simulink model "simulink_elevation_model"  (R2021b)
settings: Solver=FixedStepAuto  StartTime=0.0  StopTime=6  RelTol=1e-3
values from neighbouring files (symbols this model uses):
  fric_gear_motor = 0.0226    [loading_project.m]
  fric_gear_turrent_gun = 100/(185)    (= 0.540540540541)    [loading_project.m]
  ts3 = 10^-3    (= 0.001)    [loading_project.m]
libraries: simulink x4, dspsrcs4 x1
(part 1 of 2)
settings Model: Creator=noait  LastModifiedBy=noait

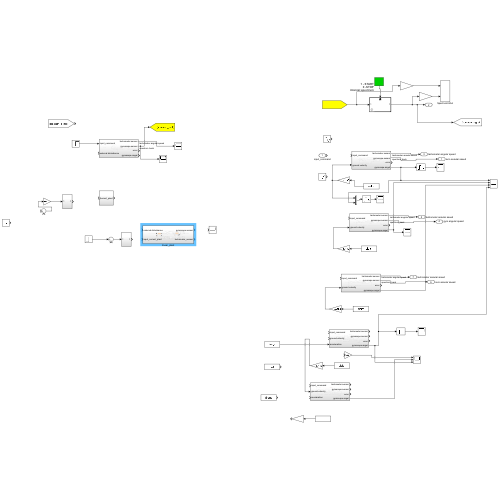
[thumbnail: Simulink's stored preview of the top-level diagram]
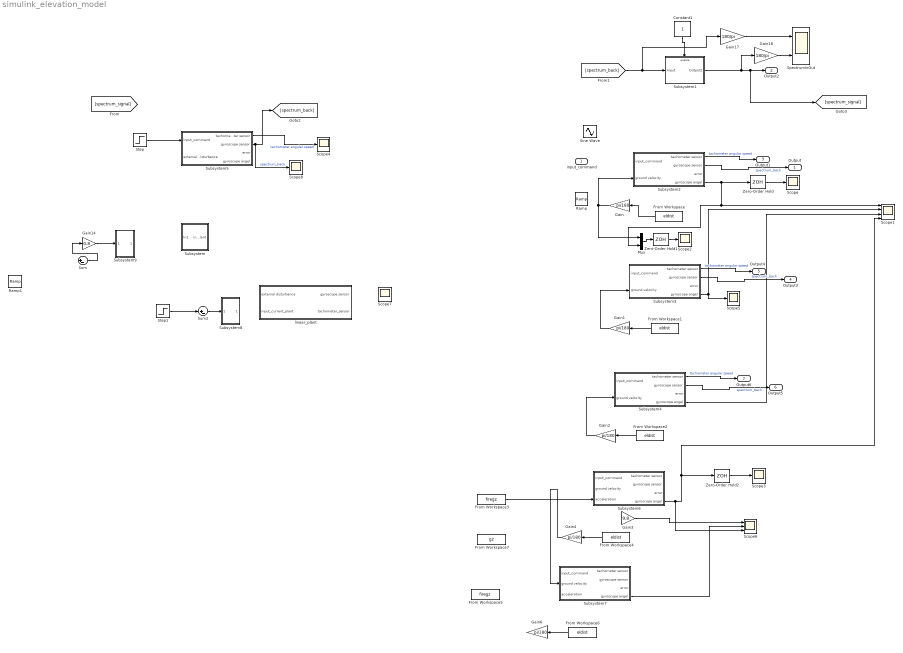
== system simulink_elevation_model ==
  input_command : Inport
  Constant1 : Constant  OutDataTypeStr=boolean
      settings: AttributesFormatString=1 - START\n0 -STOP\ninternal spectrum
      settings: OpenFcn=|
      | if get_param(gcbh,'value')-48 set_param(gcbh,'value','0','backgroundcolor','red');
      | else set_param(gcbh,'value','1','backgroundcolor','green');
      | end
  From Workspace{,1..2,4,6} (5 alike) : FromWorkspace  VariableName=eldist  SampleTime=-1  Interpolate=off  ZeroCross=off  OutputAfterFinalValue=Setting to zero
  From Workspace3 : FromWorkspace  VariableName=firegz  SampleTime=-1  OutputAfterFinalValue=Setting to zero
  From Workspace5 : FromWorkspace  VariableName=firegz  SampleTime=-1  OutputAfterFinalValue=Setting to zero
  From Workspace7 : FromWorkspace  VariableName=gz  SampleTime=ts3/3
  Gain{,1..2,4,6} (5 alike) : Gain  Gain=pi/180
  Gain14 : Gain  Gain=0.8
  Gain17 : Gain  Gain=180/pi
  Gain18 : Gain  Gain=180/pi
  Gain3 : Gain  Gain=9.8
  Mux : Mux  Inputs=2
  Ramp : simulink/Sources/Ramp  slope=1  start=0  InitialOutput=0
  Ramp1 : simulink/Sources/Ramp  slope=1  start=0  InitialOutput=0
  Scope{,2..5,7..8} (7 alike) : Scope
  Scope1 : Scope  NumInputPorts=4
  Scope6 : Scope  NumInputPorts=3
  Sine Wave : Sin  Amplitude=0.05  Frequency=2*pi  SampleTime=0
  SpectrumInOut : Scope  NumInputPorts=2
  Step : Step  After=0.05  SampleTime=0  VectorParams1D=off  ZeroCross=off
  Step1 : Step  SampleTime=0  ZeroCross=off
  Subsystem : Subsystem
  Subsystem1 : Subsystem  mask{GAIN=0.05%2*pi/180%0.5*pi/180, InitFreq=1, TargetTime=500, FreqAtTime=500}
      mask prompts: InitFreq "INITIAL FREQUENCY"; TargetTime "Target Time"; FreqAtTime "Frequency at Time"
  Subsystem2 : Subsystem
  Subsystem3 : Subsystem
  Subsystem4 : Subsystem
  Subsystem5 : Subsystem
  Subsystem6 : Subsystem
  Subsystem7 : Subsystem
  Subsystem8 : Subsystem
  Subsystem9 : Subsystem
  Sum : Sum  Inputs=|+-
  Sum2 : Sum  Inputs=|+-
  Zero-Order Hold : ZeroOrderHold  SampleTime=-1
  Zero-Order Hold1 : ZeroOrderHold  SampleTime=-1
  Zero-Order Hold2 : ZeroOrderHold  SampleTime=-1
  linear_plant : Subsystem  Description=elevation-plant
  Output : Outport  SignalName=gyro angular speed
  Output2 : Outport  Port=2
  Output1 : Outport  Port=3  SignalName=tachometer angular speed
  Output3 : Outport  Port=4  SignalName=gyro angular speed
  Output4 : Outport  Port=5  SignalName=tachometer angular speed
  Output5 : Outport  Port=6  SignalName=gyro angular speed
  Output6 : Outport  Port=7  SignalName=tachometer angular speed
  wires:
  Subsystem2/1(tachometer sensor) -> Output1/1  "tachometer angular speed"
  Gain18/1 -> SpectrumInOut/2
  Subsystem1/1(Output2) -> [spectrum_signal], Output2/1, Gain18/1
  Gain17/1 -> SpectrumInOut/1
  [spectrum_back] -> Gain17/1, Subsystem1/1(Input)
  Subsystem2/2(gyroscope sensor) -> Output/1  "spectrum_back"
  Constant1/1 -> Subsystem1/Enable
  Gain/1 -> Subsystem2/2(ground velocity), Mux/1
  Subsystem3/2(gyroscope sensor) -> Output3/1  "spectrum_back"
  From Workspace1/1 -> Gain1/1
  Gain1/1 -> Subsystem3/2(ground velocity)
  Subsystem3/1(tachometer sensor) -> Output4/1  "tachometer angular speed"
  Subsystem3/4(gyroscope angel) -> Scope5/1, Scope1/2
  Subsystem4/1(tachometer sensor) -> Output6/1  "tachometer angular speed"
  From Workspace2/1 -> Gain2/1
  Gain2/1 -> Subsystem4/2(ground velocity)
  Subsystem4/2(gyroscope sensor) -> Output5/1  "spectrum_back"
  Subsystem4/4(gyroscope angel) -> Scope1/3
  From Workspace/1 -> Gain/1
  Subsystem2/4(gyroscope angel) -> Zero-Order Hold/1, Mux/2, Scope1/1
  Zero-Order Hold/1 -> Scope/1
  Zero-Order Hold1/1 -> Scope2/1
  Mux/1 -> Zero-Order Hold1/1
  From Workspace4/1 -> Gain4/1
  Gain3/1 -> Scope6/1
  Subsystem7/4(gyroscope angel) -> Scope6/2
  From Workspace6/1 -> Gain6/1
  Sum/1 -> Gain14/1
  Gain14/1 -> Subsystem9/1(In1)
  Zero-Order Hold2/1 -> Scope3/1
  Subsystem6/4(gyroscope angel) -> Scope6/3, Zero-Order Hold2/1, Scope1/4
  Subsystem5/1(tachometer sensor) -> Scope4/1  "tachometer angular speed"
  Gain4/1 -> Subsystem7/2(ground velocity)
  From Workspace3/1 -> Subsystem6/3(acceleration)
  Sum2/1 -> Subsystem8/1(In1)
  Step1/1 -> Sum2/1
  Step/1 -> Subsystem5/1(input_command)
  Subsystem5/2(gyroscope sensor) -> Scope8/1, [spectrum_back]  "spectrum_back"

== system simulink_elevation_model/Subsystem ==
  In1 : Inport
  Gain : Gain  Gain=4.5
  Gain1 : Gain
  Gain2 : Gain  Gain=1.8*2*pi
  Integrator : Integrator
  Sum : Sum  Inputs=|++
  Transfer Fcn1 : TransferFcn  Numerator=[1 21 1.806*10^4]  Denominator=[1 25.035 2.102*10^4]
  Transfer Fcn10 : TransferFcn  Numerator=[1 59.495 9.908*10^4]  Denominator=[1 40 8.72*10^4]
  Transfer Fcn7 : TransferFcn  Denominator=[1/(2*pi*6.38)^2 0.55/355 1]
  Transfer Fcn8 : TransferFcn  Numerator=[1 2*0.08*2*35.6*pi (2*pi*35.6)^2]  Denominator=[1 2*0.94*2*35.6*pi (2*pi*35.6)^2]
  input_current_plant : Outport
  wires:
  In1/1 -> Transfer Fcn7/1
  Transfer Fcn8/1 -> Gain/1
  Transfer Fcn7/1 -> Transfer Fcn10/1
  Transfer Fcn10/1 -> Transfer Fcn1/1
  Transfer Fcn1/1 -> Transfer Fcn8/1
  Gain/1 -> Gain1/1, Gain2/1
  Integrator/1 -> Sum/1
  Gain2/1 -> Integrator/1
  Sum/1 -> input_current_plant/1
  Gain1/1 -> Sum/2

== system simulink_elevation_model/Subsystem1 ==
  Input : Inport
  Enable : EnablePort  StatesWhenEnabling=reset
  Chirp : dspsrcs4/Chirp  sweep=Linear  mode=Unidirectional  f0=1  f1=160  t1=160  Tsweep=160  phase=0  Ts=1/1000  spf=1  datatype=Double  OutputFrames=off
  Chirp Signal : simulink/Sources/Chirp Signal  Commented=on  f1=InitFreq  T=TargetTime  f2=FreqAtTime
  Chirp Signal1 : simulink/Sources/Chirp Signal  f1=1  T=160  f2=160
  Mux2 : Mux  Inputs=2
  Scope2 : Scope
  TSABAD_out_log : Scope
  gain 3 : Gain  Gain=GAIN  SaturateOnIntegerOverflow=on  SampleTime=ts3/9  OutDataTypeStr=Inherit: Same as input  ParamDataTypeStr=Inherit: Same as input
  Output2 : Outport
  wires:
  gain 3/1 -> Output2/1, Mux2/1
  Chirp Signal/1 -> ?
  Input/1 -> Mux2/2
  Mux2/1 -> TSABAD_out_log/1
  Chirp Signal1/1 -> gain 3/1, Scope2/1

== system simulink_elevation_model/Subsystem2 ==
  note: FEEDFORWARD GROUND DISTRIBUTION
  note: current
  note: gyro
  note: tachometer
  note: simple
      | controller
      | gyro
  note: controller tacho
  note: controller gyro
  input_command : Inport
  ground velocity : Inport  Port=2
  Constant : Constant  Value=0
  Gain14 : Gain  Gain=0.8
  Integrator : Integrator
  Manual Switch : ManualSwitch  CurrentSetting=0
  Subsystem1 : Subsystem
  Subsystem2 : Subsystem
  Sum : Sum  Inputs=-+|
  Sum4 : Sum  Inputs=|+-
  Transfer Fcn : TransferFcn  Numerator=[0.003753 0.1609 350.7 0]  Denominator=[0.001592 1.064 178.8 8.72*10^4]
  close loop or open loop : ManualSwitch  CurrentSetting=0
  controller or without : ManualSwitch  CurrentSetting=0
  gyro or tacho : ManualSwitch  CurrentSetting=0
  plant : Subsystem  Description=elevation-plant
  tachometer sensor : Outport
  gyroscope sensor : Outport  Port=2
  error : Outport  Port=3
  gyroscope angel : Outport  Port=4
  wires:
  Sum4/1 -> Subsystem2/1(In1), controller or without/1, error/1, Gain14/1
  Gain14/1 -> Subsystem1/1(In1)
  input_command/1 -> Sum4/1
  Subsystem1/1(Output) -> gyro or tacho/2
  Subsystem2/1(Out1) -> gyro or tacho/1
  ground velocity/1 -> Transfer Fcn/1, plant/1(external disturbance)  "ground_distribution_velocity"
  plant/1(gyroscope sensor) -> Manual Switch/2, Integrator/1, gyroscope sensor/1
  plant/2(tachometer sensor) -> Manual Switch/1, tachometer sensor/1
  Sum/1 -> plant/2(input current plant)
  gyro or tacho/1 -> controller or without/2
  controller or without/1 -> Sum/2
  Manual Switch/1 -> close loop or open loop/2
  Constant/1 -> close loop or open loop/1
  close loop or open loop/1 -> Sum4/2
  Integrator/1 -> gyroscope angel/1
  Transfer Fcn/1 -> Sum/1

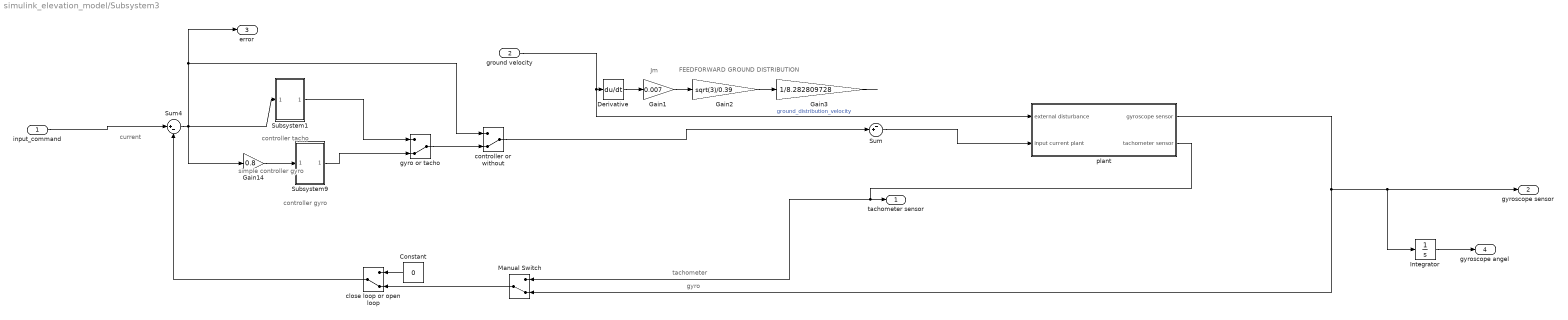
== system simulink_elevation_model/Subsystem3 ==
  note: FEEDFORWARD GROUND DISTRIBUTION
  note: Jm
  note: current
  note: gyro
  note: tachometer
  note: simple
      | controller
      | gyro
  note: controller tacho
  note: controller gyro
  input_command : Inport
  ground velocity : Inport  Port=2
  Constant : Constant  Value=0
  Derivative : Derivative
  Gain1 : Gain  Gain=0.007
  Gain14 : Gain  Gain=0.8
  Gain2 : Gain  Gain=sqrt(3)/0.39
  Gain3 : Gain  Gain=1/8.282809728
  Integrator : Integrator
  Manual Switch : ManualSwitch  CurrentSetting=0
  Subsystem1 : Subsystem
  Subsystem9 : Subsystem
  Sum : Sum  Inputs=-+|
  Sum4 : Sum  Inputs=|+-
  close loop or open loop : ManualSwitch  CurrentSetting=0
  controller or without : ManualSwitch  CurrentSetting=0
  gyro or tacho : ManualSwitch  CurrentSetting=0
  plant : Subsystem  Description=elevation-plant
  tachometer sensor : Outport
  gyroscope sensor : Outport  Port=2
  error : Outport  Port=3
  gyroscope angel : Outport  Port=4
  wires:
  Sum4/1 -> Subsystem1/1(In1), controller or without/1, error/1, Gain14/1
  Gain14/1 -> Subsystem9/1(In1)
  input_command/1 -> Sum4/1
  Subsystem9/1(Output) -> gyro or tacho/2
  Subsystem1/1(Out1) -> gyro or tacho/1
  ground velocity/1 -> Derivative/1, plant/1(external disturbance)  "ground_distribution_velocity"
  plant/1(gyroscope sensor) -> Manual Switch/2, Integrator/1, gyroscope sensor/1
  plant/2(tachometer sensor) -> Manual Switch/1, tachometer sensor/1
  Sum/1 -> plant/2(input current plant)
  Derivative/1 -> Gain1/1
  Gain1/1 -> Gain2/1
  Gain2/1 -> Gain3/1
  gyro or tacho/1 -> controller or without/2
  controller or without/1 -> Sum/2
  Manual Switch/1 -> close loop or open loop/2
  Constant/1 -> close loop or open loop/1
  close loop or open loop/1 -> Sum4/2
  Integrator/1 -> gyroscope angel/1
  Gain3/1 -> ?

== system simulink_elevation_model/Subsystem4 ==
  note: FEEDFORWARD GROUND DISTRIBUTION
  note: Jm
  note: current
  note: gyro
  note: tachometer
  note: simple
      | controller
      | gyro
  note: controller tacho
  note: controller gyro
  input_command : Inport
  ground velocity : Inport  Port=2
  Constant : Constant  Value=0
  Derivative : Derivative
  Gain1 : Gain  Gain=0.007
  Gain14 : Gain  Gain=0.8
  Gain2 : Gain  Gain=sqrt(3)/0.39
  Gain3 : Gain  Gain=1/8.282809728
  Integrator : Integrator
  Manual Switch : ManualSwitch  CurrentSetting=0
  Subsystem2 : Subsystem
  Subsystem9 : Subsystem
  Sum : Sum  Inputs=-+|
  Sum4 : Sum  Inputs=|+-
  close loop or open loop : ManualSwitch  CurrentSetting=0
  controller or without : ManualSwitch  CurrentSetting=0
  gyro or tacho : ManualSwitch  CurrentSetting=0
  plant : Subsystem  Description=elevation-plant
  tachometer sensor : Outport
  gyroscope sensor : Outport  Port=2
  error : Outport  Port=3
  gyroscope angel : Outport  Port=4
  wires:
  Sum4/1 -> Subsystem2/1(In1), controller or without/1, error/1, Gain14/1
  Gain14/1 -> Subsystem9/1(In1)
  input_command/1 -> Sum4/1
  Subsystem9/1(Output) -> gyro or tacho/2
  Subsystem2/1(Out1) -> gyro or tacho/1
  ground velocity/1 -> Derivative/1, plant/1(external disturbance)  "ground_distribution_velocity"
  plant/1(gyroscope sensor) -> Manual Switch/2, Integrator/1, gyroscope sensor/1
  plant/2(tachometer sensor) -> Manual Switch/1, tachometer sensor/1
  Sum/1 -> plant/2(input current plant)
  Derivative/1 -> Gain1/1
  Gain1/1 -> Gain2/1
  Gain2/1 -> Gain3/1
  gyro or tacho/1 -> controller or without/2
  controller or without/1 -> Sum/2
  Manual Switch/1 -> close loop or open loop/2
  Constant/1 -> close loop or open loop/1
  close loop or open loop/1 -> Sum4/2
  Integrator/1 -> gyroscope angel/1
  Gain3/1 -> ?

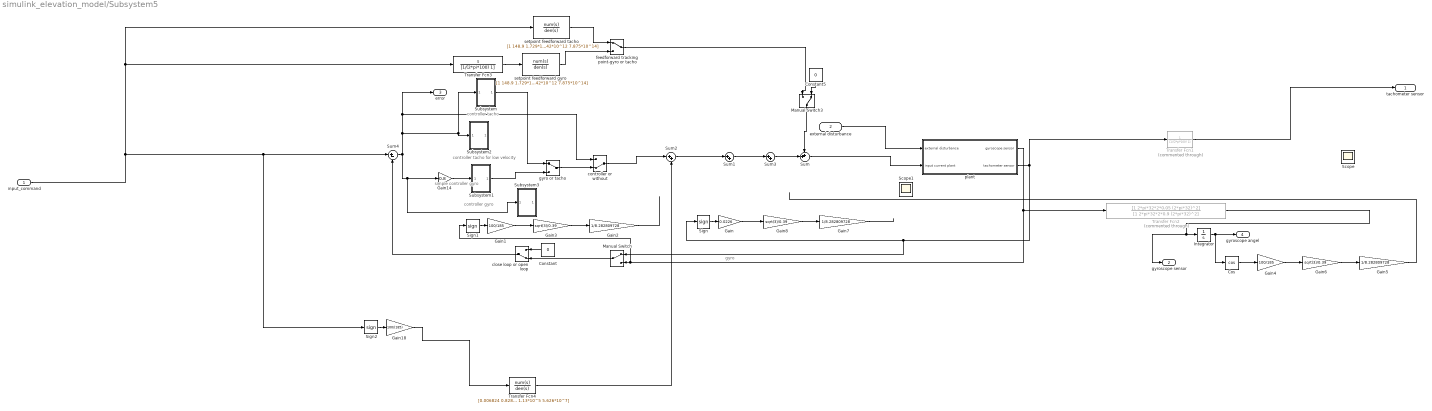
== system simulink_elevation_model/Subsystem5 ==
  note: controller tacho for low velocity
  note: gyro
  note: simple
      | controller
      | gyro
  note: controller tacho
  note: controller gyro
  input_command : Inport
  external disturbance : Inport  Port=2
  Constant : Constant  Value=0
  Constant5 : Constant  Value=0
  Cos : Trigonometry  Operator=cos
  Gain : Gain  Gain=0.0226
  Gain1 : Gain  Gain=100/185
  Gain14 : Gain  Gain=0.8
  Gain18 : Gain  Gain=100/(185)
  Gain2 : Gain  Gain=1/8.282809728
  Gain3 : Gain  Gain=sqrt(3)/0.39
  Gain4 : Gain  Gain=100/185
  Gain5 : Gain  Gain=1/8.282809728
  Gain6 : Gain  Gain=sqrt(3)/0.39
  Gain7 : Gain  Gain=1/8.282809728
  Gain8 : Gain  Gain=sqrt(3)/0.39
  Integrator : Integrator
  Manual Switch : ManualSwitch
  Manual Switch3 : ManualSwitch  CurrentSetting=0
  Scope : Scope
  Scope1 : Scope
  Sign : Signum
  Sign1 : Signum
  Sign2 : Signum
  Subsystem : Subsystem
  Subsystem1 : Subsystem
  Subsystem2 : Subsystem
  Subsystem3 : Subsystem
  Sum : Sum  Inputs=++|
  Sum1 : Sum  Inputs=|++
  Sum2 : Sum  Inputs=|++
  Sum3 : Sum  Inputs=|++
  Sum4 : Sum  Inputs=|+-
  Transfer Fcn1 : TransferFcn  Commented=through  Denominator=[1/(2*pi*100) 1]
  Transfer Fcn2 : TransferFcn  Commented=through  Numerator=[1 2*pi*32*2*0.05 (2*pi*32)^2]  Denominator=[1 2*pi*32*2*0.9 (2*pi*32)^2]
  Transfer Fcn3 : TransferFcn  Numerator=[1 0]  Denominator=[1/(2*pi*100) 1]
  Transfer Fcn4 : TransferFcn  Numerator=[0.006824 0.8287 1005 6.059*10^4 3.016*10^7]  Denominator="[0.0001 1  685.1 1.13*10^5 5.626*10^7]"
  close loop or open loop : ManualSwitch  CurrentSetting=0
  controller or without : ManualSwitch  CurrentSetting=0
  feedforward tracking point-gyro or tacho : ManualSwitch
  gyro or tacho : ManualSwitch
  plant : Subsystem  Description=elevation-plant
  setpoint feedforward gyro : TransferFcn  Numerator=[1 148.9 1.729*10^5 1.52*10^7 7.802*10^9 2.769*10^11 8.762*10^13 ]  Denominator="[2.319 3072  1.316*10^6 3.383*10^8 9.734*10^10 3.742*10^12 7.875*10^14]"
  setpoint feedforward tacho : TransferFcn  Numerator=[1 148.9 1.729*10^5 1.52*10^7 7.802*10^9 2.769*10^11 8.762*10^13 0]  Denominator=[0.424 295 6.504*10^4 3.101*10^7 1.76*10^9 5.413*10^11 3.742*10^12 7.875*10^14]
  tachometer sensor : Outport
  gyroscope sensor : Outport  Port=2
  error : Outport  Port=3
  gyroscope angel : Outport  Port=4
  wires:
  Gain14/1 -> Subsystem1/1(In1)
  gyro or tacho/1 -> controller or without/2
  Manual Switch/1 -> close loop or open loop/2
  Constant/1 -> close loop or open loop/1
  Integrator/1 -> Cos/1, gyroscope angel/1
  setpoint feedforward gyro/1 -> feedforward tracking point-gyro or tacho/2
  feedforward tracking point-gyro or tacho/1 -> Manual Switch3/1
  Sum4/1 -> Subsystem/1(In1), Subsystem2/1(In1), error/1, controller or without/1, Subsystem3/1(In1), Gain14/1
  Constant5/1 -> Manual Switch3/2
  Manual Switch3/1 -> Sum/1
  ? -> ?
  Transfer Fcn3/1 -> setpoint feedforward gyro/1
  Sign/1 -> Gain/1
  Gain8/1 -> Gain7/1
  Gain/1 -> Gain8/1
  Gain7/1 -> ?
  Gain3/1 -> Gain2/1
  Gain1/1 -> Gain3/1
  Sign1/1 -> Gain1/1
  controller or without/1 -> Sum2/1
  Sum2/1 -> Sum1/1
  Sum1/1 -> Sum3/1
  Sum3/1 -> Sum/2
  close loop or open loop/1 -> Sum4/2
  external disturbance/1 -> plant/1(external disturbance)
  plant/1(gyroscope sensor) -> Sign1/1, Manual Switch/2, Transfer Fcn2/1
  Transfer Fcn2/1 -> gyroscope sensor/1, Integrator/1
  plant/2(tachometer sensor) -> Manual Switch/1, Sign/1, Transfer Fcn1/1
  input_command/1 -> Sign2/1, Sum4/1, Transfer Fcn3/1, setpoint feedforward tacho/1
  Sum/1 -> plant/2(input current plant)
  Gain2/1 -> ?
  Transfer Fcn1/1 -> tachometer sensor/1
  setpoint feedforward tacho/1 -> feedforward tracking point-gyro or tacho/1
  Subsystem1/1(Output) -> gyro or tacho/2
  Subsystem/1(Out1) -> gyro or tacho/1
  Gain4/1 -> Gain6/1
  Gain6/1 -> Gain5/1
  Cos/1 -> Gain4/1
  Gain5/1 -> ?
  Gain18/1 -> Transfer Fcn4/1
  Sign2/1 -> Gain18/1
  Transfer Fcn4/1 -> Sum2/2

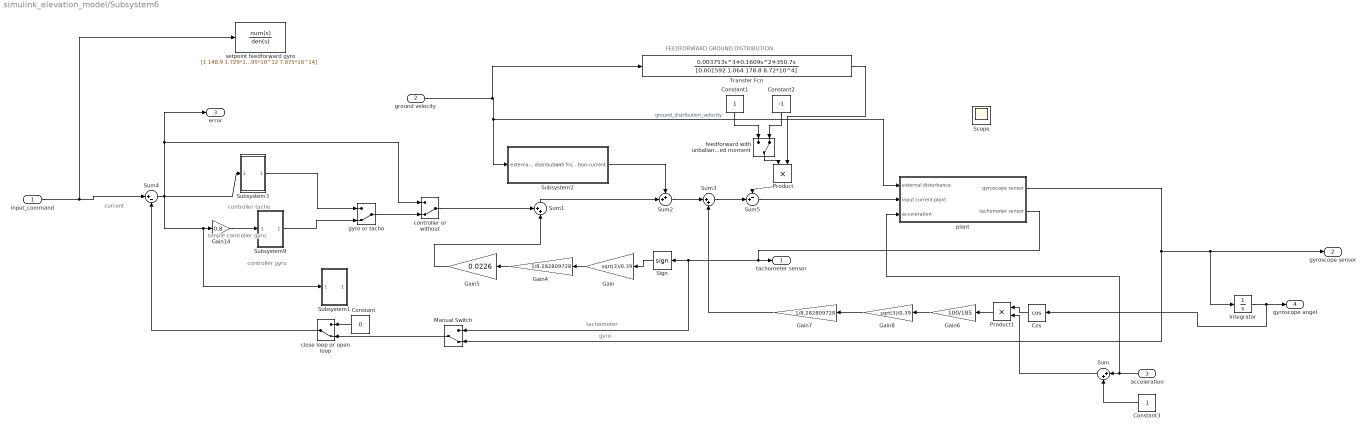
== system simulink_elevation_model/Subsystem6 ==
  note: FEEDFORWARD GROUND DISTRIBUTION
  note: current
  note: gyro
  note: tachometer
  note: simple
      | controller
      | gyro
  note: controller tacho
  note: controller gyro
  input_command : Inport
  ground velocity : Inport  Port=2
  acceleration : Inport  Port=3
  Constant : Constant  Value=0
  Constant1 : Constant
  Constant2 : Constant  Value=-1
  Constant3 : Constant
  Cos : Trigonometry  Operator=cos
  Gain : Gain  Gain=sqrt(3)/0.39
  Gain14 : Gain  Gain=0.8
  Gain4 : Gain  Gain=1/8.282809728
  Gain5 : Gain  Gain=0.0226
  Gain6 : Gain  Gain=100/185
  Gain7 : Gain  Gain=1/8.282809728
  Gain8 : Gain  Gain=sqrt(3)/0.39
  Integrator : Integrator
  Manual Switch : ManualSwitch  CurrentSetting=0
  Product : Product
  Product1 : Product
  Scope : Scope
  Sign : Signum
  Subsystem1 : Subsystem
  Subsystem2 : Subsystem
  Subsystem3 : Subsystem
  Subsystem9 : Subsystem
  Sum : Sum  Inputs=|++
  Sum1 : Sum  Inputs=++|
  Sum2 : Sum  Inputs=++|
  Sum3 : Sum  Inputs=|++
  Sum4 : Sum  Inputs=|+-
  Sum5 : Sum  Inputs=-+|
  Transfer Fcn : TransferFcn  Numerator="[0.003753 0.1609 350.7  0]"  Denominator=[0.001592 1.064 178.8 8.72*10^4]
  close loop or open loop : ManualSwitch  CurrentSetting=0
  controller or without : ManualSwitch  CurrentSetting=0
  feedforward with unballanced moment : ManualSwitch  CurrentSetting=0
  gyro or tacho : ManualSwitch  CurrentSetting=0
  plant : Subsystem  Description=elevation-plant
  setpoint feedforward gyro : TransferFcn  Numerator=[1 148.9 1.729*10^5 1.52*10^7 7.802*10^9 2.769*10^11 8.762*10^13 0]  Denominator=[0.003691 7.208 5167 1.855*10^6 4.932*10^8 1.033*10^11 4.995*10^12 7.875*10^14]
  tachometer sensor : Outport
  gyroscope sensor : Outport  Port=2
  error : Outport  Port=3
  gyroscope angel : Outport  Port=4
  wires:
  Sum4/1 -> Subsystem3/1(In1), controller or without/1, error/1, Subsystem1/1(In1), Gain14/1
  Gain14/1 -> Subsystem9/1(In1)
  Subsystem3/1(Out1) -> gyro or tacho/1
  ground velocity/1 -> Transfer Fcn/1, Subsystem2/1(external distribution), plant/1(external disturbance)  "ground_distribution_velocity"
  plant/1(gyroscope sensor) -> Manual Switch/2, Integrator/1, gyroscope sensor/1
  plant/2(tachometer sensor) -> Sign/1, Manual Switch/1, tachometer sensor/1
  gyro or tacho/1 -> controller or without/2
  Manual Switch/1 -> close loop or open loop/2
  Constant/1 -> close loop or open loop/1
  close loop or open loop/1 -> Sum4/2
  Integrator/1 -> Cos/1, gyroscope angel/1
  Sign/1 -> Gain/1
  Gain/1 -> Gain4/1
  Gain4/1 -> Gain5/1
  Gain5/1 -> Sum1/2
  controller or without/1 -> Sum1/1
  Sum1/1 -> Sum2/2
  input_command/1 -> setpoint feedforward gyro/1, Sum4/1
  Sum2/1 -> Sum3/1
  Gain8/1 -> Gain7/1
  Gain6/1 -> Gain8/1
  Sum3/1 -> Sum5/2
  Subsystem2/1(anti friction current) -> Sum2/1
  Gain7/1 -> Sum3/2
  Constant2/1 -> feedforward with unballanced moment/2
  Constant1/1 -> feedforward with unballanced moment/1
  feedforward with unballanced moment/1 -> Product/1
  Product/1 -> Sum5/1
  Sum5/1 -> plant/2(input current plant)
  Cos/1 -> Product1/1
  Product1/1 -> Gain6/1
  acceleration/1 -> plant/3(acceleration), Sum/1
  Constant3/1 -> Sum/2
  Sum/1 -> Product1/2
  Transfer Fcn/1 -> Product/2
  Subsystem9/1(Output) -> gyro or tacho/2

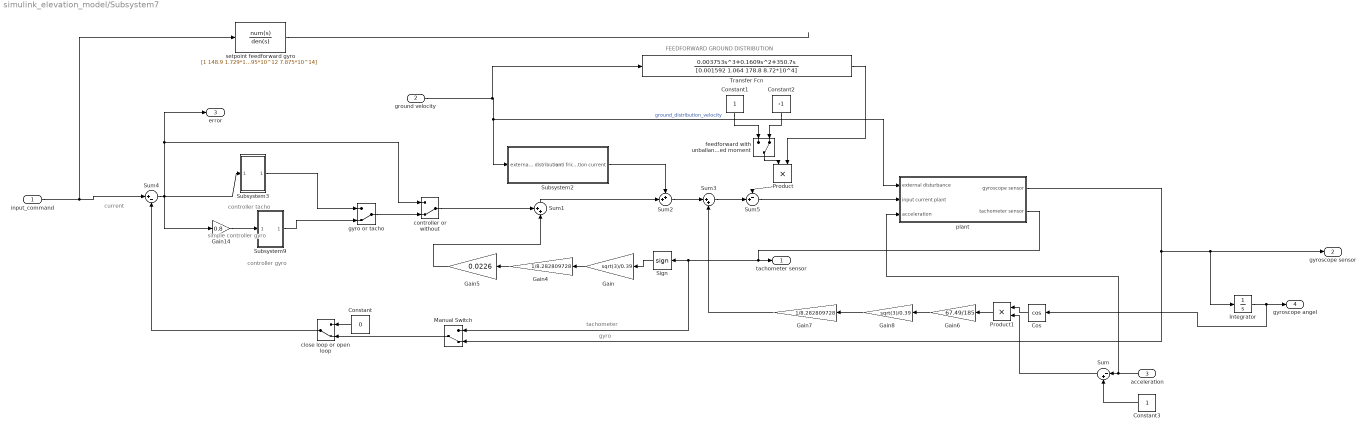
== system simulink_elevation_model/Subsystem7 ==
  note: FEEDFORWARD GROUND DISTRIBUTION
  note: current
  note: gyro
  note: tachometer
  note: simple
      | controller
      | gyro
  note: controller tacho
  note: controller gyro
  input_command : Inport
  ground velocity : Inport  Port=2
  acceleration : Inport  Port=3
  Constant : Constant  Value=0
  Constant1 : Constant
  Constant2 : Constant  Value=-1
  Constant3 : Constant
  Cos : Trigonometry  Operator=cos
  Gain : Gain  Gain=sqrt(3)/0.39
  Gain14 : Gain  Gain=0.8
  Gain4 : Gain  Gain=1/8.282809728
  Gain5 : Gain  Gain=0.0226
  Gain6 : Gain  Gain=67.49/185
  Gain7 : Gain  Gain=1/8.282809728
  Gain8 : Gain  Gain=sqrt(3)/0.39
  Integrator : Integrator
  Manual Switch : ManualSwitch  CurrentSetting=0
  Product : Product
  Product1 : Product
  Sign : Signum
  Subsystem2 : Subsystem
  Subsystem3 : Subsystem
  Subsystem9 : Subsystem
  Sum : Sum  Inputs=|-+
  Sum1 : Sum  Inputs=++|
  Sum2 : Sum  Inputs=++|
  Sum3 : Sum  Inputs=|++
  Sum4 : Sum  Inputs=|+-
  Sum5 : Sum  Inputs=-+|
  Transfer Fcn : TransferFcn  Numerator="[0.003753 0.1609 350.7  0]"  Denominator=[0.001592 1.064 178.8 8.72*10^4]
  close loop or open loop : ManualSwitch  CurrentSetting=0
  controller or without : ManualSwitch  CurrentSetting=0
  feedforward with unballanced moment : ManualSwitch  CurrentSetting=0
  gyro or tacho : ManualSwitch  CurrentSetting=0
  plant : Subsystem  Description=elevation-plant
  setpoint feedforward gyro : TransferFcn  Numerator=[1 148.9 1.729*10^5 1.52*10^7 7.802*10^9 2.769*10^11 8.762*10^13 0]  Denominator=[0.003691 7.208 5167 1.855*10^6 4.932*10^8 1.033*10^11 4.995*10^12 7.875*10^14]
  tachometer sensor : Outport
  gyroscope sensor : Outport  Port=2
  error : Outport  Port=3
  gyroscope angel : Outport  Port=4
  wires:
  Sum4/1 -> Subsystem3/1(In1), controller or without/1, error/1, Gain14/1
  Gain14/1 -> Subsystem9/1(In1)
  Subsystem9/1(Output) -> gyro or tacho/2
  Subsystem3/1(Out1) -> gyro or tacho/1
  ground velocity/1 -> Transfer Fcn/1, Subsystem2/1(external distribution), plant/1(external disturbance)  "ground_distribution_velocity"
  plant/1(gyroscope sensor) -> Manual Switch/2, Integrator/1, gyroscope sensor/1
  plant/2(tachometer sensor) -> Sign/1, Manual Switch/1, tachometer sensor/1
  gyro or tacho/1 -> controller or without/2
  Manual Switch/1 -> close loop or open loop/2
  Constant/1 -> close loop or open loop/1
  close loop or open loop/1 -> Sum4/2
  Integrator/1 -> Cos/1, gyroscope angel/1
  Sign/1 -> Gain/1
  Gain/1 -> Gain4/1
  Gain4/1 -> Gain5/1
  Gain5/1 -> Sum1/2
  controller or without/1 -> Sum1/1
  Sum1/1 -> Sum2/2
  input_command/1 -> setpoint feedforward gyro/1, Sum4/1
  Sum2/1 -> Sum3/1
  Gain8/1 -> Gain7/1
  Gain6/1 -> Gain8/1
  Sum3/1 -> Sum5/2
  Subsystem2/1(anti friction current) -> Sum2/1
  Gain7/1 -> Sum3/2
  Constant2/1 -> feedforward with unballanced moment/2
  Constant1/1 -> feedforward with unballanced moment/1
  feedforward with unballanced moment/1 -> Product/1
  Transfer Fcn/1 -> Product/2
  Product/1 -> Sum5/1
  setpoint feedforward gyro/1 -> ?
  Sum5/1 -> plant/2(input current plant)
  Cos/1 -> Product1/1
  Product1/1 -> Gain6/1
  acceleration/1 -> plant/3(acceleration), Sum/1
  Constant3/1 -> Sum/2
  Sum/1 -> Product1/2

== system simulink_elevation_model/Subsystem8 ==
  In1 : Inport
  Gain : Gain  Gain=1.6
  Gain1 : Gain  Gain=50
  Integrator : Integrator
  Sum : Sum  Inputs=|++
  Transfer Fcn1 : TransferFcn  Numerator=[1 59.49 9.908*10^4]  Denominator=[1 40 8.72*10^4]
  Transfer Fcn2 : TransferFcn  Numerator=[0.016 1]  Denominator=[0.008 1]
  Transfer Fcn4 : TransferFcn  Numerator=[1 21 1.806*10^4]  Denominator=[1 11.06 9607]
  Transfer Fcn5 : TransferFcn  Numerator=[1 16.78 (2*pi*36)^2]  Denominator=[1 188.3 (2*pi*36)^2]
  Output : Outport
  wires:
  Transfer Fcn5/1 -> Transfer Fcn4/1
  Integrator/1 -> Sum/1
  Gain1/1 -> Integrator/1
  Gain/1 -> Sum/2
  Transfer Fcn4/1 -> Gain/1, Gain1/1
  Sum/1 -> Output/1
  Transfer Fcn1/1 -> Transfer Fcn5/1
  Transfer Fcn2/1 -> Transfer Fcn1/1
  In1/1 -> Transfer Fcn2/1

== system simulink_elevation_model/Subsystem9 ==
  In1 : Inport
  Gain : Gain  Gain=10
  Gain1 : Gain  Gain=26
  Integrator : Integrator
  Sum : Sum  Inputs=|++
  Transfer Fcn4 : TransferFcn  Numerator=[1 2*pi*21.3*2*0.05 (2*pi*21.3)^2]  Denominator=[1 2*pi*21.3*2*0.48 (2*pi*21.3)^2]
  Transfer Fcn5 : TransferFcn  Numerator=[1 16.78 (2*pi*36)^2]  Denominator=[1 188.3 (2*pi*36)^2]
  Output : Outport
  wires:
  Transfer Fcn5/1 -> Transfer Fcn4/1
  In1/1 -> Transfer Fcn5/1
  Integrator/1 -> Sum/1
  Gain1/1 -> Integrator/1
  Gain/1 -> Sum/2
  Transfer Fcn4/1 -> Gain/1, Gain1/1
  Sum/1 -> Output/1

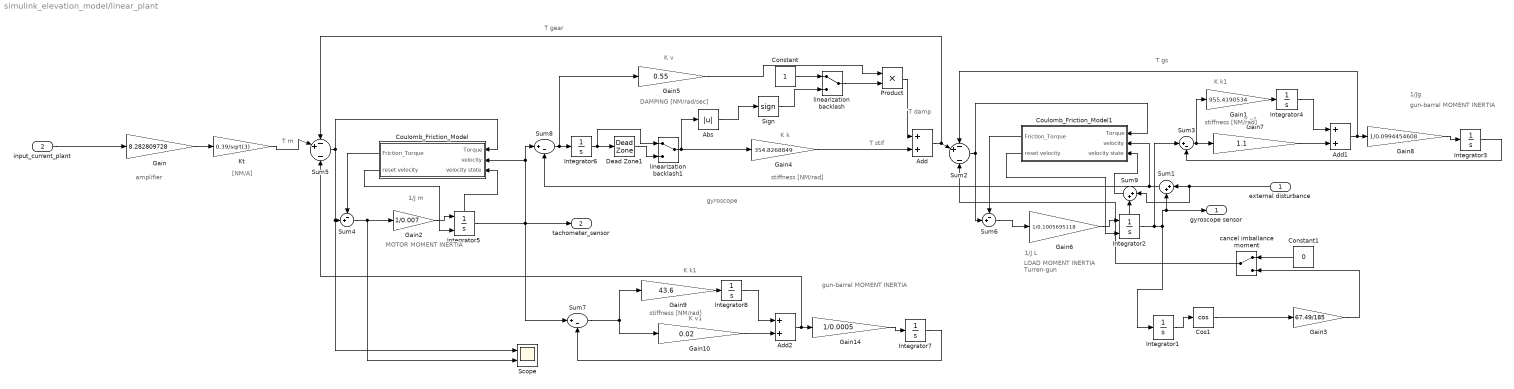
== system simulink_elevation_model/linear_plant ==
  note: T gs
  note: [NM/A]
  note: K v
  note: amplifier
  note: DAMPING
      | [NM/rad/sec]
  note: K k1
  note: T damp
  note: K v1
  note: stiffness
      | [NM/rad]
  note: 1/J m
  note: MOTOR
      | MOMENT INERTIA
  note: T m
  note: 1/J L
  note: T stif
  note: K k
  note: T gear
  note: LOAD
      | MOMENT INERTIA
      | Turren-gun
  note: stiffness
      | [NM/rad]
  note: gyroscope
  note: gun-barral
      | MOMENT INERTIA
  note: 1/Jg
  note: K v1
  note: K k1
  note: stiffness
      | [NM/rad]
  note: gun-barral
      | MOMENT INERTIA
  external disturbance : Inport
  input_current_plant : Inport  Port=2
  Abs : Abs
  Add : Sum
  Add1 : Sum
  Add2 : Sum
  Constant : Constant
  Constant1 : Constant  Value=0
  Cos1 : Trigonometry  Operator=cos
  Coulomb_Friction_Model : Subsystem
  Coulomb_Friction_Model1 : Subsystem
  Dead Zone1 : DeadZone  LowerValue=-0.07*10^-3  UpperValue=0.07*10^-3  ZeroCross=off
  Gain : Gain  Gain=8.282809728
  Gain1 : Gain  Gain=955.4190534
  Gain10 : Gain  Gain=0.02
  Gain14 : Gain  Gain=1/0.0005
  Gain2 : Gain  Gain=1/0.007
  Gain3 : Gain  Gain=67.49/185
  Gain4 : Gain  Gain=354.8268849
  Gain5 : Gain  Gain=0.55
  Gain6 : Gain  Gain=1/0.1005695118
  Gain7 : Gain  Gain=1.1
  Gain8 : Gain  Gain=1/0.0994454608
  Gain9 : Gain  Gain=43.6
  Integrator1 : Integrator  UpperSaturationLimit=pi/2  LowerSaturationLimit=0  WrappedStateUpperValue=pi/2  WrappedStateLowerValue=0
  Integrator2 : Integrator  ExternalReset=rising  ShowStatePort=on  ZeroCross=off
  Integrator{3..4,6..8} (5 alike) : Integrator
  Integrator5 : Integrator  ExternalReset=rising  ShowStatePort=on  ZeroCross=off
  Kt : Gain  Gain=0.39/sqrt(3)
  Product : Product
  Scope : Scope  NumInputPorts=2
  Sign : Signum
  Sum1 : Sum  Inputs=|++
  Sum2 : Sum  Inputs=-+|-
  Sum3 : Sum  Inputs=|+-
  Sum4 : Sum  Inputs=-+|
  Sum5 : Sum  Inputs=-+|-
  Sum6 : Sum  Inputs=-+|
  Sum7 : Sum  Inputs=|+-
  Sum8 : Sum  Inputs=|+-
  Sum9 : Sum  Inputs=|++
  cancel imballance moment : ManualSwitch
  linearization backlash : ManualSwitch
  linearization backlash1 : ManualSwitch
  gyroscope sensor : Outport
  tachometer_sensor : Outport  Port=2
  wires:
  Constant/1 -> linearization backlash/1
  Gain/1 -> Kt/1
  Add/1 -> Sum5/1, Sum2/2
  Integrator4/1 -> Add1/1
  Kt/1 -> Sum5/2
  Gain6/1 -> Integrator2/1
  Gain5/1 -> Product/1
  Gain4/1 -> Add/2
  Sum3/1 -> Gain7/1, Gain1/1
  Sum8/1 -> Gain5/1, Integrator6/1
  Gain2/1 -> Integrator5/1
  Product/1 -> Add/1
  Integrator6/1 -> linearization backlash1/1, Dead Zone1/1
  Abs/1 -> Sign/1
  Gain7/1 -> Add1/2
  linearization backlash/1 -> Product/2
  Integrator3/1 -> Sum3/2
  Sign/1 -> linearization backlash/2
  Gain1/1 -> Integrator4/1
  Sum4/1 -> Scope/2, Gain2/1
  Sum5/1 -> Coulomb_Friction_Model/1(Torque), Scope/1, Sum4/2
  Sum6/1 -> Gain6/1
  Gain8/1 -> Integrator3/1
  Add1/1 -> Gain8/1, Sum2/1
  Integrator2/1 -> Sum3/1, Integrator1/1, Sum1/2, gyroscope sensor/1
  input_current_plant/1 -> Gain/1
  Sum2/1 -> Sum6/2, Coulomb_Friction_Model1/1(Torque)
  Coulomb_Friction_Model/1(Friction_Torque) -> Sum4/1
  Integrator5/State -> Coulomb_Friction_Model/3(velocity state)
  Coulomb_Friction_Model/2(reset velocity) -> Integrator5/2
  Integrator1/1 -> Cos1/1
  Integrator8/1 -> Add2/1
  Gain9/1 -> Integrator8/1
  Gain10/1 -> Add2/2
  Gain14/1 -> Integrator7/1
  Add2/1 -> Sum5/3, Gain14/1
  Sum7/1 -> Gain10/1, Gain9/1
  Integrator7/1 -> Sum7/2
  Cos1/1 -> Gain3/1
  linearization backlash1/1 -> Abs/1, Gain4/1
  Gain3/1 -> cancel imballance moment/2
  cancel imballance moment/1 -> Sum2/3
  Constant1/1 -> cancel imballance moment/1
  Dead Zone1/1 -> linearization backlash1/2
  Coulomb_Friction_Model1/1(Friction_Torque) -> Sum6/1
  Coulomb_Friction_Model1/2(reset velocity) -> Integrator2/2
  Sum1/1 -> Coulomb_Friction_Model1/2(velocity), Sum8/2
  Integrator2/State -> Sum9/2
  Sum9/1 -> Coulomb_Friction_Model1/3(velocity state)
  Integrator5/1 -> tachometer_sensor/1, Sum7/1, Coulomb_Friction_Model/2(velocity), Sum8/1
  external disturbance/1 -> Sum9/1, Sum1/1

== system simulink_elevation_model/Subsystem2/Subsystem1 ==
  In1 : Inport
  Gain : Gain  Gain=10
  Gain1 : Gain  Gain=26
  Integrator : Integrator
  Sum : Sum  Inputs=|++
  Transfer Fcn4 : TransferFcn  Numerator=[1 2*pi*21.3*2*0.05 (2*pi*21.3)^2]  Denominator=[1 2*pi*21.3*2*0.48 (2*pi*21.3)^2]
  Transfer Fcn5 : TransferFcn  Numerator=[1 16.78 (2*pi*36)^2]  Denominator=[1 188.3 (2*pi*36)^2]
  Output : Outport
  wires:
  Transfer Fcn5/1 -> Transfer Fcn4/1
  In1/1 -> Transfer Fcn5/1
  Integrator/1 -> Sum/1
  Gain1/1 -> Integrator/1
  Gain/1 -> Sum/2
  Transfer Fcn4/1 -> Gain/1, Gain1/1
  Sum/1 -> Output/1

== system simulink_elevation_model/Subsystem2/Subsystem2 ==
  In1 : Inport
  Gain : Gain  Gain=4.5
  Gain1 : Gain
  Gain2 : Gain  Gain=1.8*2*pi
  Integrator : Integrator
  Sum : Sum  Inputs=|++
  Transfer Fcn1 : TransferFcn  Numerator=[1 21 1.806*10^4]  Denominator=[1 25.035 2.102*10^4]
  Transfer Fcn10 : TransferFcn  Numerator=[1 59.495 9.908*10^4]  Denominator=[1 40 8.72*10^4]
  Transfer Fcn7 : TransferFcn  Denominator=[1/(2*pi*6.38)^2 0.55/355 1]
  Transfer Fcn8 : TransferFcn  Numerator=[1 2*0.08*2*35.6*pi (2*pi*35.6)^2]  Denominator=[1 2*0.94*2*35.6*pi (2*pi*35.6)^2]
  Out1 : Outport
  wires:
  Gain/1 -> Gain1/1, Gain2/1
  Sum/1 -> Out1/1
  In1/1 -> Transfer Fcn7/1
  Transfer Fcn8/1 -> Gain/1
  Transfer Fcn7/1 -> Transfer Fcn10/1
  Transfer Fcn10/1 -> Transfer Fcn1/1
  Transfer Fcn1/1 -> Transfer Fcn8/1
  Gain2/1 -> Integrator/1
  Gain1/1 -> Sum/2
  Integrator/1 -> Sum/1

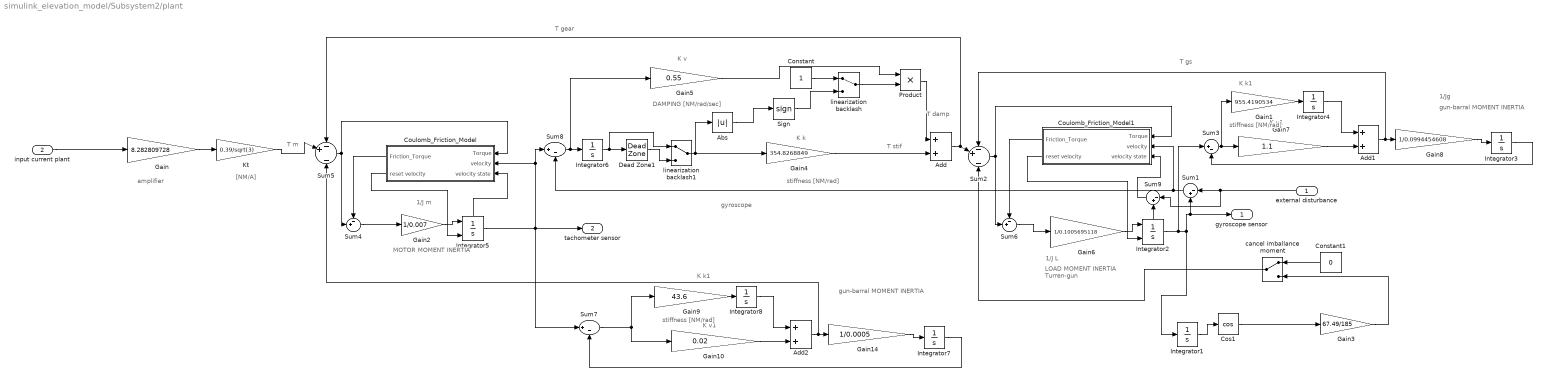
== system simulink_elevation_model/Subsystem2/plant ==
  note: T gs
  note: [NM/A]
  note: K v
  note: amplifier
  note: DAMPING
      | [NM/rad/sec]
  note: K k1
  note: T damp
  note: K v1
  note: stiffness
      | [NM/rad]
  note: 1/J m
  note: MOTOR
      | MOMENT INERTIA
  note: T m
  note: 1/J L
  note: T stif
  note: K k
  note: T gear
  note: LOAD
      | MOMENT INERTIA
      | Turren-gun
  note: stiffness
      | [NM/rad]
  note: gyroscope
  note: gun-barral
      | MOMENT INERTIA
  note: 1/Jg
  note: K v1
  note: K k1
  note: stiffness
      | [NM/rad]
  note: gun-barral
      | MOMENT INERTIA
  external disturbance : Inport
  input current plant : Inport  Port=2
  Abs : Abs
  Add : Sum
  Add1 : Sum
  Add2 : Sum
  Constant : Constant
  Constant1 : Constant  Value=0
  Cos1 : Trigonometry  Operator=cos
  Coulomb_Friction_Model : Subsystem
  Coulomb_Friction_Model1 : Subsystem
  Dead Zone1 : DeadZone  LowerValue=-0.07*10^-3  UpperValue=0.07*10^-3  ZeroCross=off
  Gain : Gain  Gain=8.282809728
  Gain1 : Gain  Gain=955.4190534
  Gain10 : Gain  Gain=0.02
  Gain14 : Gain  Gain=1/0.0005
  Gain2 : Gain  Gain=1/0.007
  Gain3 : Gain  Gain=67.49/185
  Gain4 : Gain  Gain=354.8268849
  Gain5 : Gain  Gain=0.55
  Gain6 : Gain  Gain=1/0.1005695118
  Gain7 : Gain  Gain=1.1
  Gain8 : Gain  Gain=1/0.0994454608
  Gain9 : Gain  Gain=43.6
  Integrator1 : Integrator  UpperSaturationLimit=pi/2  LowerSaturationLimit=0  WrappedStateUpperValue=pi/2  WrappedStateLowerValue=0
  Integrator2 : Integrator  ExternalReset=rising  ShowStatePort=on  ZeroCross=off
  Integrator{3..4,6..8} (5 alike) : Integrator
  Integrator5 : Integrator  ExternalReset=rising  ShowStatePort=on  ZeroCross=off
  Kt : Gain  Gain=0.39/sqrt(3)
  Product : Product
  Sign : Signum
  Sum1 : Sum  Inputs=|-+
  Sum2 : Sum  Inputs=-+|-
  Sum3 : Sum  Inputs=|+-
  Sum4 : Sum  Inputs=-+|
  Sum5 : Sum  Inputs=-+|-
  Sum6 : Sum  Inputs=-+|
  Sum7 : Sum  Inputs=|+-
  Sum8 : Sum  Inputs=|+-
  Sum9 : Sum  Inputs=|-+
  cancel imballance moment : ManualSwitch
  linearization backlash : ManualSwitch
  linearization backlash1 : ManualSwitch
  gyroscope sensor : Outport
  tachometer sensor : Outport  Port=2
  wires:
  Constant/1 -> linearization backlash/1
  Gain/1 -> Kt/1
  Add/1 -> Sum2/2, Sum5/1
  Integrator4/1 -> Add1/1
  Kt/1 -> Sum5/2
  Gain6/1 -> Integrator2/1
  Gain5/1 -> Product/1
  Gain4/1 -> Add/2
  Sum3/1 -> Gain7/1, Gain1/1
  Sum8/1 -> Gain5/1, Integrator6/1
  Gain2/1 -> Integrator5/1
  Product/1 -> Add/1
  Integrator6/1 -> linearization backlash1/1, Dead Zone1/1
  Abs/1 -> Sign/1
  Gain7/1 -> Add1/2
  linearization backlash/1 -> Product/2
  Integrator3/1 -> Sum3/2
  Sign/1 -> linearization backlash/2
  Gain1/1 -> Integrator4/1
  Sum4/1 -> Gain2/1
  Sum5/1 -> Coulomb_Friction_Model/1(Torque), Sum4/2
  Sum6/1 -> Gain6/1
  Gain8/1 -> Integrator3/1
  Add1/1 -> Gain8/1, Sum2/1
  Integrator2/1 -> Sum3/1, Integrator1/1, Sum1/2, gyroscope sensor/1
  input current plant/1 -> Gain/1
  Sum2/1 -> Sum6/2, Coulomb_Friction_Model1/1(Torque)
  Coulomb_Friction_Model/1(Friction_Torque) -> Sum4/1
  Integrator5/State -> Coulomb_Friction_Model/3(velocity state)
  Coulomb_Friction_Model/2(reset velocity) -> Integrator5/2
  Integrator1/1 -> Cos1/1
  Integrator8/1 -> Add2/1
  Gain9/1 -> Integrator8/1
  Gain10/1 -> Add2/2
  Gain14/1 -> Integrator7/1
  Add2/1 -> Sum5/3, Gain14/1
  Sum7/1 -> Gain10/1, Gain9/1
  Integrator7/1 -> Sum7/2
  Cos1/1 -> Gain3/1
  linearization backlash1/1 -> Abs/1, Gain4/1
  Gain3/1 -> cancel imballance moment/2
  cancel imballance moment/1 -> Sum2/3
  Constant1/1 -> cancel imballance moment/1
  Dead Zone1/1 -> linearization backlash1/2
  Coulomb_Friction_Model1/1(Friction_Torque) -> Sum6/1
  Coulomb_Friction_Model1/2(reset velocity) -> Integrator2/2
  Sum1/1 -> Coulomb_Friction_Model1/2(velocity), Sum8/2
  Integrator2/State -> Sum9/2
  Sum9/1 -> Coulomb_Friction_Model1/3(velocity state)
  Integrator5/1 -> tachometer sensor/1, Sum7/1, Coulomb_Friction_Model/2(velocity), Sum8/1
  external disturbance/1 -> Sum9/1, Sum1/1

== system simulink_elevation_model/Subsystem3/Subsystem1 ==
  In1 : Inport
  Gain : Gain  Gain=4.5
  Gain1 : Gain
  Gain2 : Gain  Gain=1.8*2*pi
  Integrator : Integrator
  Sum : Sum  Inputs=|++
  Transfer Fcn1 : TransferFcn  Numerator=[1 21 1.806*10^4]  Denominator=[1 25.035 2.102*10^4]
  Transfer Fcn10 : TransferFcn  Numerator=[1 59.495 9.908*10^4]  Denominator=[1 40 8.72*10^4]
  Transfer Fcn7 : TransferFcn  Denominator=[1/(2*pi*6.38)^2 0.55/355 1]
  Transfer Fcn8 : TransferFcn  Numerator=[1 2*0.08*2*35.6*pi (2*pi*35.6)^2]  Denominator=[1 2*0.94*2*35.6*pi (2*pi*35.6)^2]
  Out1 : Outport
  wires:
  Gain/1 -> Gain1/1, Gain2/1
  Sum/1 -> Out1/1
  In1/1 -> Transfer Fcn7/1
  Transfer Fcn8/1 -> Gain/1
  Transfer Fcn7/1 -> Transfer Fcn10/1
  Transfer Fcn10/1 -> Transfer Fcn1/1
  Transfer Fcn1/1 -> Transfer Fcn8/1
  Gain2/1 -> Integrator/1
  Gain1/1 -> Sum/2
  Integrator/1 -> Sum/1

== system simulink_elevation_model/Subsystem3/Subsystem9 ==
  In1 : Inport
  Gain : Gain  Gain=10
  Gain1 : Gain  Gain=26
  Integrator : Integrator
  Sum : Sum  Inputs=|++
  Transfer Fcn4 : TransferFcn  Numerator=[1 2*pi*21.3*2*0.05 (2*pi*21.3)^2]  Denominator=[1 2*pi*21.3*2*0.48 (2*pi*21.3)^2]
  Transfer Fcn5 : TransferFcn  Numerator=[1 16.78 (2*pi*36)^2]  Denominator=[1 188.3 (2*pi*36)^2]
  Output : Outport
  wires:
  Transfer Fcn5/1 -> Transfer Fcn4/1
  In1/1 -> Transfer Fcn5/1
  Integrator/1 -> Sum/1
  Gain1/1 -> Integrator/1
  Gain/1 -> Sum/2
  Transfer Fcn4/1 -> Gain/1, Gain1/1
  Sum/1 -> Output/1

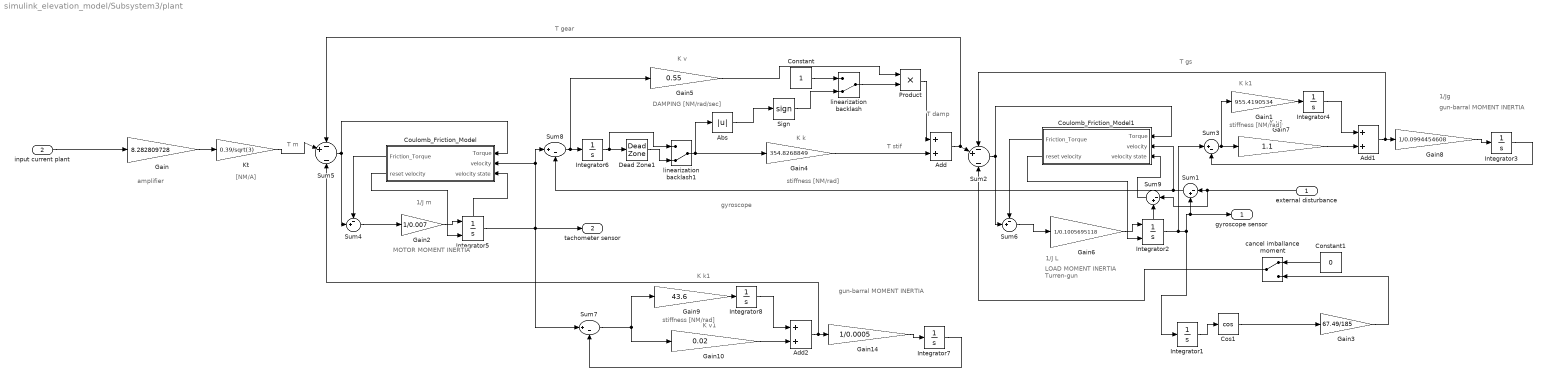
== system simulink_elevation_model/Subsystem3/plant ==
  note: T gs
  note: [NM/A]
  note: K v
  note: amplifier
  note: DAMPING
      | [NM/rad/sec]
  note: K k1
  note: T damp
  note: K v1
  note: stiffness
      | [NM/rad]
  note: 1/J m
  note: MOTOR
      | MOMENT INERTIA
  note: T m
  note: 1/J L
  note: T stif
  note: K k
  note: T gear
  note: LOAD
      | MOMENT INERTIA
      | Turren-gun
  note: stiffness
      | [NM/rad]
  note: gyroscope
  note: gun-barral
      | MOMENT INERTIA
  note: 1/Jg
  note: K v1
  note: K k1
  note: stiffness
      | [NM/rad]
  note: gun-barral
      | MOMENT INERTIA
  external disturbance : Inport
  input current plant : Inport  Port=2
  Abs : Abs
  Add : Sum
  Add1 : Sum
  Add2 : Sum
  Constant : Constant
  Constant1 : Constant  Value=0
  Cos1 : Trigonometry  Operator=cos
  Coulomb_Friction_Model : Subsystem
  Coulomb_Friction_Model1 : Subsystem
  Dead Zone1 : DeadZone  LowerValue=-0.07*10^-3  UpperValue=0.07*10^-3  ZeroCross=off
  Gain : Gain  Gain=8.282809728
  Gain1 : Gain  Gain=955.4190534
  Gain10 : Gain  Gain=0.02
  Gain14 : Gain  Gain=1/0.0005
  Gain2 : Gain  Gain=1/0.007
  Gain3 : Gain  Gain=67.49/185
  Gain4 : Gain  Gain=354.8268849
  Gain5 : Gain  Gain=0.55
  Gain6 : Gain  Gain=1/0.1005695118
  Gain7 : Gain  Gain=1.1
  Gain8 : Gain  Gain=1/0.0994454608
  Gain9 : Gain  Gain=43.6
  Integrator1 : Integrator  UpperSaturationLimit=pi/2  LowerSaturationLimit=0  WrappedStateUpperValue=pi/2  WrappedStateLowerValue=0
  Integrator2 : Integrator  ExternalReset=rising  ShowStatePort=on  ZeroCross=off
  Integrator{3..4,6..8} (5 alike) : Integrator
  Integrator5 : Integrator  ExternalReset=rising  ShowStatePort=on  ZeroCross=off
  Kt : Gain  Gain=0.39/sqrt(3)
  Product : Product
  Sign : Signum
  Sum1 : Sum  Inputs=|-+
  Sum2 : Sum  Inputs=-+|-
  Sum3 : Sum  Inputs=|+-
  Sum4 : Sum  Inputs=-+|
  Sum5 : Sum  Inputs=-+|-
  Sum6 : Sum  Inputs=-+|
  Sum7 : Sum  Inputs=|+-
  Sum8 : Sum  Inputs=|+-
  Sum9 : Sum  Inputs=|-+
  cancel imballance moment : ManualSwitch
  linearization backlash : ManualSwitch  CurrentSetting=0
  linearization backlash1 : ManualSwitch  CurrentSetting=0
  gyroscope sensor : Outport
  tachometer sensor : Outport  Port=2
  wires:
  Constant/1 -> linearization backlash/1
  Gain/1 -> Kt/1
  Add/1 -> Sum2/2, Sum5/1
  Integrator4/1 -> Add1/1
  Kt/1 -> Sum5/2
  Gain6/1 -> Integrator2/1
  Gain5/1 -> Product/1
  Gain4/1 -> Add/2
  Sum3/1 -> Gain7/1, Gain1/1
  Sum8/1 -> Gain5/1, Integrator6/1
  Gain2/1 -> Integrator5/1
  Product/1 -> Add/1
  Integrator6/1 -> linearization backlash1/1, Dead Zone1/1
  Abs/1 -> Sign/1
  Gain7/1 -> Add1/2
  linearization backlash/1 -> Product/2
  Integrator3/1 -> Sum3/2
  Sign/1 -> linearization backlash/2
  Gain1/1 -> Integrator4/1
  Sum4/1 -> Gain2/1
  Sum5/1 -> Coulomb_Friction_Model/1(Torque), Sum4/2
  Sum6/1 -> Gain6/1
  Gain8/1 -> Integrator3/1
  Add1/1 -> Gain8/1, Sum2/1
  Integrator2/1 -> Sum3/1, Integrator1/1, Sum1/2, gyroscope sensor/1
  input current plant/1 -> Gain/1
  Sum2/1 -> Sum6/2, Coulomb_Friction_Model1/1(Torque)
  Coulomb_Friction_Model/1(Friction_Torque) -> Sum4/1
  Integrator5/State -> Coulomb_Friction_Model/3(velocity state)
  Coulomb_Friction_Model/2(reset velocity) -> Integrator5/2
  Integrator1/1 -> Cos1/1
  Integrator8/1 -> Add2/1
  Gain9/1 -> Integrator8/1
  Gain10/1 -> Add2/2
  Gain14/1 -> Integrator7/1
  Add2/1 -> Sum5/3, Gain14/1
  Sum7/1 -> Gain10/1, Gain9/1
  Integrator7/1 -> Sum7/2
  Cos1/1 -> Gain3/1
  linearization backlash1/1 -> Abs/1, Gain4/1
  Gain3/1 -> cancel imballance moment/2
  cancel imballance moment/1 -> Sum2/3
  Constant1/1 -> cancel imballance moment/1
  Dead Zone1/1 -> linearization backlash1/2
  Coulomb_Friction_Model1/1(Friction_Torque) -> Sum6/1
  Coulomb_Friction_Model1/2(reset velocity) -> Integrator2/2
  external disturbance/1 -> Sum9/1, Sum1/1
  Sum1/1 -> Coulomb_Friction_Model1/2(velocity), Sum8/2
  Integrator2/State -> Sum9/2
  Sum9/1 -> Coulomb_Friction_Model1/3(velocity state)
  Integrator5/1 -> tachometer sensor/1, Sum7/1, Coulomb_Friction_Model/2(velocity), Sum8/1

== system simulink_elevation_model/Subsystem4/Subsystem2 ==
  In1 : Inport
  Gain : Gain  Gain=4.5
  Gain1 : Gain
  Gain2 : Gain  Gain=1.8*2*pi
  Integrator : Integrator
  Sum : Sum  Inputs=|++
  Transfer Fcn1 : TransferFcn  Numerator=[1 21 1.806*10^4]  Denominator=[1 25.035 2.102*10^4]
  Transfer Fcn10 : TransferFcn  Numerator=[1 59.495 9.908*10^4]  Denominator=[1 40 8.72*10^4]
  Transfer Fcn7 : TransferFcn  Denominator=[1/(2*pi*6.38)^2 0.55/355 1]
  Transfer Fcn8 : TransferFcn  Numerator=[1 2*0.08*2*35.6*pi (2*pi*35.6)^2]  Denominator=[1 2*0.94*2*35.6*pi (2*pi*35.6)^2]
  Out1 : Outport
  wires:
  Gain/1 -> Gain1/1, Gain2/1
  Sum/1 -> Out1/1
  In1/1 -> Transfer Fcn7/1
  Transfer Fcn8/1 -> Gain/1
  Transfer Fcn7/1 -> Transfer Fcn10/1
  Transfer Fcn10/1 -> Transfer Fcn1/1
  Transfer Fcn1/1 -> Transfer Fcn8/1
  Gain2/1 -> Integrator/1
  Gain1/1 -> Sum/2
  Integrator/1 -> Sum/1

== system simulink_elevation_model/Subsystem4/Subsystem9 ==
  In1 : Inport
  Gain : Gain  Gain=10
  Gain1 : Gain  Gain=26
  Integrator : Integrator
  Sum : Sum  Inputs=|++
  Transfer Fcn4 : TransferFcn  Numerator=[1 2*pi*21.3*2*0.05 (2*pi*21.3)^2]  Denominator=[1 2*pi*21.3*2*0.48 (2*pi*21.3)^2]
  Transfer Fcn5 : TransferFcn  Numerator=[1 16.78 (2*pi*36)^2]  Denominator=[1 188.3 (2*pi*36)^2]
  Output : Outport
  wires:
  Transfer Fcn5/1 -> Transfer Fcn4/1
  In1/1 -> Transfer Fcn5/1
  Integrator/1 -> Sum/1
  Gain1/1 -> Integrator/1
  Gain/1 -> Sum/2
  Transfer Fcn4/1 -> Gain/1, Gain1/1
  Sum/1 -> Output/1

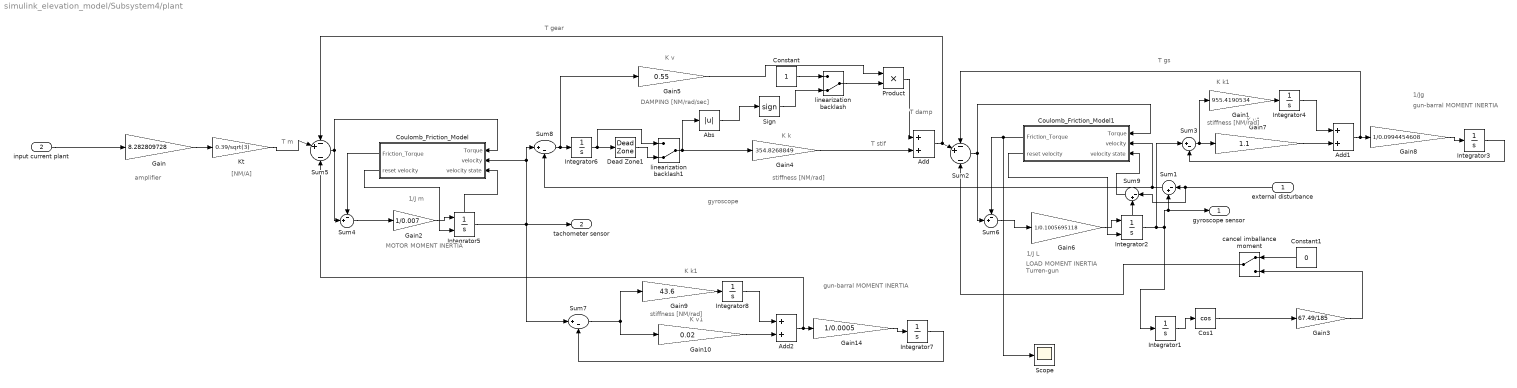
== system simulink_elevation_model/Subsystem4/plant ==
  note: T gs
  note: [NM/A]
  note: K v
  note: amplifier
  note: DAMPING
      | [NM/rad/sec]
  note: K k1
  note: T damp
  note: K v1
  note: stiffness
      | [NM/rad]
  note: 1/J m
  note: MOTOR
      | MOMENT INERTIA
  note: T m
  note: 1/J L
  note: T stif
  note: K k
  note: T gear
  note: LOAD
      | MOMENT INERTIA
      | Turren-gun
  note: stiffness
      | [NM/rad]
  note: gyroscope
  note: gun-barral
      | MOMENT INERTIA
  note: 1/Jg
  note: K v1
  note: K k1
  note: stiffness
      | [NM/rad]
  note: gun-barral
      | MOMENT INERTIA
  external disturbance : Inport
  input current plant : Inport  Port=2
  Abs : Abs
  Add : Sum
  Add1 : Sum
  Add2 : Sum
  Constant : Constant
  Constant1 : Constant  Value=0
  Cos1 : Trigonometry  Operator=cos
  Coulomb_Friction_Model : Subsystem
  Coulomb_Friction_Model1 : Subsystem
  Dead Zone1 : DeadZone  LowerValue=-0.07*10^-3  UpperValue=0.07*10^-3  ZeroCross=off
  Gain : Gain  Gain=8.282809728
  Gain1 : Gain  Gain=955.4190534
  Gain10 : Gain  Gain=0.02
  Gain14 : Gain  Gain=1/0.0005
  Gain2 : Gain  Gain=1/0.007
  Gain3 : Gain  Gain=67.49/185
  Gain4 : Gain  Gain=354.8268849
  Gain5 : Gain  Gain=0.55
  Gain6 : Gain  Gain=1/0.1005695118
  Gain7 : Gain  Gain=1.1
  Gain8 : Gain  Gain=1/0.0994454608
  Gain9 : Gain  Gain=43.6
  Integrator1 : Integrator  UpperSaturationLimit=pi/2  LowerSaturationLimit=0  WrappedStateUpperValue=pi/2  WrappedStateLowerValue=0
  Integrator2 : Integrator  ExternalReset=rising  ShowStatePort=on  ZeroCross=off
  Integrator{3..4,6..8} (5 alike) : Integrator
  Integrator5 : Integrator  ExternalReset=rising  ShowStatePort=on  ZeroCross=off
  Kt : Gain  Gain=0.39/sqrt(3)
  Product : Product
  Scope : Scope
  Sign : Signum
  Sum1 : Sum  Inputs=|-+
  Sum2 : Sum  Inputs=-+|-
  Sum3 : Sum  Inputs=|+-
  Sum4 : Sum  Inputs=-+|
  Sum5 : Sum  Inputs=-+|-
  Sum6 : Sum  Inputs=-+|
  Sum7 : Sum  Inputs=|+-
  Sum8 : Sum  Inputs=|+-
  Sum9 : Sum  Inputs=|-+
  cancel imballance moment : ManualSwitch
  linearization backlash : ManualSwitch  CurrentSetting=0
  linearization backlash1 : ManualSwitch  CurrentSetting=0
  gyroscope sensor : Outport
  tachometer sensor : Outport  Port=2
  wires:
  Constant/1 -> linearization backlash/1
  Gain/1 -> Kt/1
  Add/1 -> Sum2/2, Sum5/1
  Integrator4/1 -> Add1/1
  Kt/1 -> Sum5/2
  Gain6/1 -> Integrator2/1
  Gain5/1 -> Product/1
  Gain4/1 -> Add/2
  Sum3/1 -> Gain7/1, Gain1/1
  Sum8/1 -> Gain5/1, Integrator6/1
  Gain2/1 -> Integrator5/1
  Product/1 -> Add/1
  Integrator6/1 -> linearization backlash1/1, Dead Zone1/1
  Abs/1 -> Sign/1
  Gain7/1 -> Add1/2
  linearization backlash/1 -> Product/2
  Integrator3/1 -> Sum3/2
  Sign/1 -> linearization backlash/2
  Gain1/1 -> Integrator4/1
  Sum4/1 -> Gain2/1
  Sum5/1 -> Coulomb_Friction_Model/1(Torque), Sum4/2
  Sum6/1 -> Gain6/1
  Gain8/1 -> Integrator3/1
  Add1/1 -> Gain8/1, Sum2/1
  Integrator2/1 -> Sum3/1, Integrator1/1, Sum1/2, gyroscope sensor/1
  input current plant/1 -> Gain/1
  Sum2/1 -> Sum6/2, Coulomb_Friction_Model1/1(Torque)
  Coulomb_Friction_Model/1(Friction_Torque) -> Sum4/1
  Integrator5/State -> Coulomb_Friction_Model/3(velocity state)
  Coulomb_Friction_Model/2(reset velocity) -> Integrator5/2
  Integrator1/1 -> Cos1/1
  Integrator8/1 -> Add2/1
  Gain9/1 -> Integrator8/1
  Gain10/1 -> Add2/2
  Gain14/1 -> Integrator7/1
  Add2/1 -> Sum5/3, Gain14/1
  Sum7/1 -> Gain10/1, Gain9/1
  Integrator7/1 -> Sum7/2
  Cos1/1 -> Gain3/1
  linearization backlash1/1 -> Abs/1, Gain4/1
  Gain3/1 -> cancel imballance moment/2
  cancel imballance moment/1 -> Sum2/3
  Constant1/1 -> cancel imballance moment/1
  Dead Zone1/1 -> linearization backlash1/2
  Coulomb_Friction_Model1/1(Friction_Torque) -> Sum6/1, Scope/1
  Coulomb_Friction_Model1/2(reset velocity) -> Integrator2/2
  external disturbance/1 -> Sum9/1, Sum1/1
  Sum1/1 -> Coulomb_Friction_Model1/2(velocity), Sum8/2
  Integrator2/State -> Sum9/2
  Sum9/1 -> Coulomb_Friction_Model1/3(velocity state)
  Integrator5/1 -> tachometer sensor/1, Sum7/1, Coulomb_Friction_Model/2(velocity), Sum8/1

== system simulink_elevation_model/Subsystem5/Subsystem ==
  In1 : Inport
  Gain : Gain  Gain=4.5
  Gain1 : Gain
  Gain2 : Gain  Gain=1.8*2*pi
  Gain3 : Gain  Gain=0.3
  Integrator : Integrator
  Sum : Sum  Inputs=|+++
  Transfer Fcn : TransferFcn  Numerator=[1 0]  Denominator=[1/(2*pi*100) 1]
  Transfer Fcn1 : TransferFcn  Numerator=[1 21 1.806*10^4]  Denominator=[1 25.035 2.102*10^4]
  Transfer Fcn10 : TransferFcn  Numerator=[1 59.495 9.908*10^4]  Denominator=[1 40 8.72*10^4]
  Transfer Fcn7 : TransferFcn  Denominator=[1/(2*pi*6.38)^2 0.55/355 1]
  Transfer Fcn8 : TransferFcn  Numerator=[1 2*0.08*2*35.6*pi (2*pi*35.6)^2]  Denominator=[1 2*0.94*2*35.6*pi (2*pi*35.6)^2]
  Out1 : Outport
  wires:
  In1/1 -> Transfer Fcn7/1
  Transfer Fcn8/1 -> Gain3/1, Gain/1
  Transfer Fcn7/1 -> Transfer Fcn10/1
  Transfer Fcn10/1 -> Transfer Fcn1/1
  Transfer Fcn1/1 -> Transfer Fcn8/1
  Gain/1 -> Gain1/1, Gain2/1
  Integrator/1 -> Sum/1
  Gain2/1 -> Integrator/1
  Sum/1 -> Out1/1
  Gain1/1 -> Sum/2
  Gain3/1 -> Transfer Fcn/1
  Transfer Fcn/1 -> ?

== system simulink_elevation_model/Subsystem5/Subsystem1 ==
  In1 : Inport
  Gain : Gain  Gain=10
  Gain1 : Gain  Gain=26
  Integrator : Integrator
  Sum : Sum  Inputs=|++
  Transfer Fcn4 : TransferFcn  Numerator=[1 2*pi*21.3*2*0.05 (2*pi*21.3)^2]  Denominator=[1 2*pi*21.3*2*0.48 (2*pi*21.3)^2]
  Transfer Fcn5 : TransferFcn  Numerator=[1 16.78 (2*pi*36)^2]  Denominator=[1 188.3 (2*pi*36)^2]
  Output : Outport
  wires:
  Transfer Fcn5/1 -> Transfer Fcn4/1
  In1/1 -> Transfer Fcn5/1
  Integrator/1 -> Sum/1
  Gain1/1 -> Integrator/1
  Gain/1 -> Sum/2
  Transfer Fcn4/1 -> Gain/1, Gain1/1
  Sum/1 -> Output/1

== system simulink_elevation_model/Subsystem5/Subsystem2 ==
  In1 : Inport
  Gain : Gain  Gain=2*pi*700
  Gain1 : Gain  Gain=10
  Sum : Sum  Inputs=|++
  Transfer Fcn : TransferFcn  Denominator="[1  0]"
  Transfer Fcn10 : TransferFcn  Numerator=[1 59.495 9.908*10^4]  Denominator=[1 40 8.72*10^4]
  Out1 : Outport
  wires:
  In1/1 -> Transfer Fcn10/1
  Sum/1 -> Out1/1
  Gain1/1 -> Sum/2
  Gain/1 -> Transfer Fcn/1
  Transfer Fcn/1 -> Sum/1
  Transfer Fcn10/1 -> Gain1/1, Gain/1

== system simulink_elevation_model/Subsystem5/Subsystem3 ==
  In1 : Inport
  Gain : Gain  Gain=3
  Gain1 : Gain  Gain=100
  Integrator : Integrator
  Sum : Sum  Inputs=|++
  Transfer Fcn1 : TransferFcn  Commented=through  Numerator=[1 2*pi*32*2*0.08 (2*pi*32)^2]  Denominator=[1 2*pi*32*2*0.94 (2*pi*32)^2]
  Transfer Fcn2 : TransferFcn  Commented=through  Numerator=[1 2*pi*32*2*0.05 (2*pi*32)^2]  Denominator=[1 2*pi*32*2*0.9 (2*pi*32)^2]
  Transfer Fcn4 : TransferFcn  Commented=through  Numerator=[1 2*pi*15*2*0.5 (2*pi*15)^2]  Denominator=[1 2*pi*15*2*0.05 (2*pi*15)^2]
  Transfer Fcn5 : TransferFcn  Numerator=[1 16.78 (2*pi*36)^2]  Denominator=[1 188.3 (2*pi*36)^2]
  Output : Outport
  wires:
  Gain1/1 -> Integrator/1
  Gain/1 -> Sum/2
  Integrator/1 -> Sum/1
  Sum/1 -> Output/1
  In1/1 -> Transfer Fcn5/1
  Transfer Fcn2/1 -> Transfer Fcn1/1
  Transfer Fcn5/1 -> Transfer Fcn2/1
  Transfer Fcn1/1 -> Gain1/1, Gain/1
